simulink model "rightone"  (R2020b)
settings: Solver=VariableStepAuto  StartTime=0.0  StopTime=5  RelTol=1e-3
libraries: simulink_extras x2
settings Model: Creator=Catherina Liu  LastModifiedBy=28217

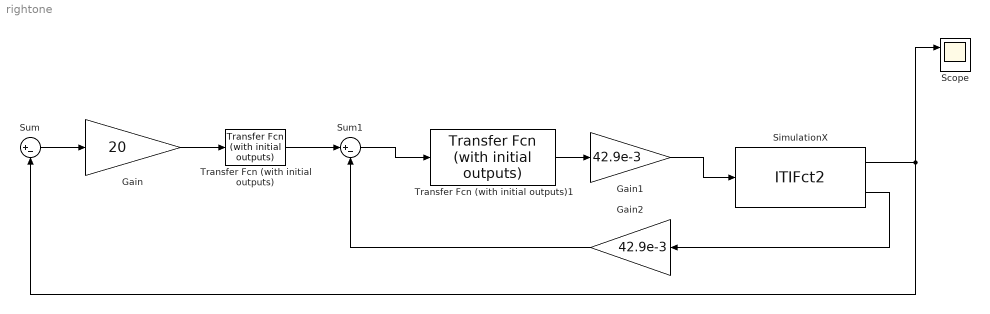
== system rightone ==
  Gain : Gain  Gain=20
  Gain1 : Gain  Gain=42.9e-3
  Gain2 : Gain  Gain=42.9e-3
  Scope : Scope  NumInputPorts=2
  "SimulationX " : S-Function  FunctionName=ITIFct2  Parameters=ip, port, ts, nIn, nOut  SFunctionDeploymentMode=off  EnableBusSupport=off  mask{ip='localhost', port=4097, ts=0.001, nIn=1, nOut=2}
      mask prompts: ip "Address: ip"; port "Port Number: port [-]"; ts "Communication Step Size: ts [s]"; nIn "Input Vector Dimension (to SimulationX): nIn [-]"; nOut "Output Vector Dimension (from SimulationX): nOut [-]"
      mask help: Coupling Element
  Sum : Sum  Inputs=|+-
  Sum1 : Sum  Inputs=|+-
  Transfer Fcn (with initial outputs) : simulink_extras/Additional Linear/Transfer Fcn (with initial outputs)  N=[5000]  D="[1  5000]"  Y0=.5  U0=0
  Transfer Fcn (with initial outputs)1 : simulink_extras/Additional Linear/Transfer Fcn (with initial outputs)  N=[1]  D="[0.514e-3  2.68]"  Y0=.5  U0=0
  wires:
  Gain/1 -> Transfer Fcn (with initial outputs)/1
  Transfer Fcn (with initial outputs)/1 -> Sum1/1
  Sum1/1 -> Transfer Fcn (with initial outputs)1/1
  Transfer Fcn (with initial outputs)1/1 -> Gain1/1
  Gain1/1 -> "SimulationX "/1
  Gain2/1 -> Sum1/2
  "SimulationX "/1 -> Scope/1, Sum/2
  Sum/1 -> Gain/1
  ? -> Scope/2, Sum/1
  "SimulationX "/2 -> Gain2/1
